simulink model "E33_VCU_simulink"  (R2014a)
settings: Solver=FixedStepDiscrete  StartTime=0.0  StopTime=10.0  FixedStep=0.0005  RelTol=1e-3
values from neighbouring files (symbols this model uses):
  Accu_FAN_Test = ecucoder_cal(Accu_FAN_Test)    [E33_VCU.m]
  Accu_FAN_threshold = ecucoder_cal(Accu_FAN_threshold)    [E33_VCU.m]
  APPS1_Voltage = ecucoder_cal(APPS1_Voltage)    [E33_VCU.m]
  APPS2_Voltage = ecucoder_cal(APPS2_Voltage)    [E33_VCU.m]
  APPS_Map = [0,1000]    [E33_VCU.m]
  APPS_threshold = ecucoder_cal(APPS_threshold)    [E33_VCU.m]
  Beep_Time = ecucoder_cal(Beep_Time)    [E33_VCU.m]
  BeeperTest = ecucoder_cal(BeeperTest)    [E33_VCU.m]
  BMSLedTest = ecucoder_cal(BMSLedTest)    [E33_VCU.m]
  BP_F_threshold = ecucoder_cal(BP_F_threshold)    [E33_VCU.m]
  BP_F_Voltage = ecucoder_cal(BP_F_Voltage)    [E33_VCU.m]
  BP_Map = [0,1000]    [E33_VCU.m]
  BP_R_Voltage = ecucoder_cal(BP_R_Voltage)    [E33_VCU.m]
  Brk_luminance = ecucoder_cal(Brk_luminance)    [E33_VCU.m]
  DCDC_Relay_Test = ecucoder_cal(DCDC_Relay_Test)    [E33_VCU.m]
  FactoryTestEnable = ecucoder_cal(FactoryTestEnable)    [E33_VCU.m]
  HardBrk_luminance = ecucoder_cal(HardBrk_luminance)    [E33_VCU.m]
  IMDLedTest = ecucoder_cal(IMDLedTest)    [E33_VCU.m]
  linear_FL_Map = ecucoder_cal(linear_FL_Map)    [E33_VCU.m]
  linear_FR_Map = ecucoder_cal(linear_FR_Map)    [E33_VCU.m]
  linear_Map = ecucoder_cal(linear_Map)    [E33_VCU.m]
  linear_RL_Map = ecucoder_cal(linear_RL_Map)    [E33_VCU.m]
  linear_RR_Map = ecucoder_cal(linear_RR_Map)    [E33_VCU.m]
  MaxPow = 40    [E33_VCU.m]
  MaxRPM = 5400    [E33_VCU.m]
  MaxRPMchangePerSec = ecucoder_cal(MaxRPMchangePerSec)    [E33_VCU.m]
  MaxTorqChangePerSec = ecucoder_cal(MaxTorqChangePerSec)    [E33_VCU.m]
  Motor_RPM_Map = (0:ceil(MaxRPM/100))*100    [E33_VCU.m]
  Pump_Test = ecucoder_cal(Pump_Test)    [E33_VCU.m]
  Pump_threshold = ecucoder_cal(Pump_threshold)    [E33_VCU.m]
  R2D_Light_Test = ecucoder_cal(R2D_Light_Test)    [E33_VCU.m]
  Radiator_FAN_Test = ecucoder_cal(Radiator_FAN_Test)    [E33_VCU.m]
  SCS_Error_5V = ecucoder_cal(SCS_Error_5V)    [E33_VCU.m]
  SCS_Error_GND = ecucoder_cal(SCS_Error_GND)    [E33_VCU.m]
  SPD_Coef = 1884/40    (= 47.1)    [E33_VCU.m]
  Tail_Light_Test = ecucoder_cal(Tail_Light_Test)    [E33_VCU.m]
  Tmanage_Map = [0,100]    [E33_VCU.m]
  Torq_percentage_Map = Motor_Torq_MAP/MaxTorq*1000    [E33_VCU.m]
libraries: simulink x164, ec55xxlib x44, dspswit3 x6
(part 3 of 5)

== system E33_VCU_simulink/Subsystem1/MCUctrl/VCU_MCU_CMD/MCU_SPD_CMD ==
  MCU_SPD_CMD : Inport
  BitCov : DataTypeConversion  OutDataTypeStr=uint8
  Constant{3..8} (6 alike) : Constant  Value=0  OutDataTypeStr=uint8  SampleTime=-1
  MCU_SPD_CMDCOV : DataTypeConversion  OutDataTypeStr=uint8
  MCU_SPD_CMDRon : Rounding  Operator=round
  MCU_SPD_CMD_1sat : Saturate  UpperLimit=65535  LowerLimit=0
  MCU_SPD_CMD_And : simulink/Logic and Bit Operations/Bitwise Operator  logicop=AND  UseBitMask=off  NumInputPorts=2  BitMask=bin2dec('11011001')  BitMaskRealWorld=Stored Integer
  MCU_SPD_CMD_And_C : Constant  Value=255  OutDataTypeStr=uint32
  MCU_SPD_CMD_Convert : DataTypeConversion  OutDataTypeStr=uint32
  MCU_SPD_CMD_D : Product  Inputs=*/
  MCU_SPD_CMD_D1 : Product  Inputs=*/
  MCU_SPD_CMD_F : Constant  Value=0.5  OutDataTypeStr=single
  MCU_SPD_CMD_L : simulink/Logic and Bit Operations/Bitwise Operator  logicop=AND  UseBitMask=on  BitMask=65535  BitMaskRealWorld=Stored Integer
  MCU_SPD_CMD_O : Constant  Value=-10000  OutDataTypeStr=single
  MCU_SPD_CMD_S : ArithShift
  MCU_SPD_CMD_sat : Saturate  UpperLimit=10000  LowerLimit=-10000
  MCU_SPD_CMD_st : Sum  Inputs=+-
  MCU_SPD_CMDoutput2_C : Constant  Value=256
  output1 : Outport
  output2 : Outport  Port=2
  output3 : Outport  Port=3
  output4 : Outport  Port=4
  output5 : Outport  Port=5
  output6 : Outport  Port=6
  output7 : Outport  Port=7
  output8 : Outport  Port=8
  wires:
  MCU_SPD_CMD/1 -> MCU_SPD_CMD_sat/1
  MCU_SPD_CMD_sat/1 -> MCU_SPD_CMD_st/1
  MCU_SPD_CMD_O/1 -> MCU_SPD_CMD_st/2
  MCU_SPD_CMD_st/1 -> MCU_SPD_CMD_D/1
  MCU_SPD_CMD_F/1 -> MCU_SPD_CMD_D/2
  MCU_SPD_CMD_D/1 -> MCU_SPD_CMDRon/1
  MCU_SPD_CMDRon/1 -> MCU_SPD_CMD_S/1
  MCU_SPD_CMD_S/1 -> MCU_SPD_CMD_1sat/1
  MCU_SPD_CMD_1sat/1 -> MCU_SPD_CMD_Convert/1
  MCU_SPD_CMD_Convert/1 -> MCU_SPD_CMD_L/1
  MCU_SPD_CMD_L/1 -> MCU_SPD_CMD_D1/1, MCU_SPD_CMD_And/1
  MCU_SPD_CMDoutput2_C/1 -> MCU_SPD_CMD_D1/2
  MCU_SPD_CMD_D1/1 -> MCU_SPD_CMDCOV/1
  MCU_SPD_CMDCOV/1 -> output2/1
  MCU_SPD_CMD_And_C/1 -> MCU_SPD_CMD_And/2
  MCU_SPD_CMD_And/1 -> BitCov/1
  BitCov/1 -> output1/1
  Constant3/1 -> output3/1
  Constant4/1 -> output4/1
  Constant5/1 -> output5/1
  Constant6/1 -> output6/1
  Constant7/1 -> output7/1
  Constant8/1 -> output8/1

== system E33_VCU_simulink/Subsystem1/MCUctrl/VCU_MCU_CMD/MCU_TORQ_CMD ==
  MCU_TORQ_CMD : Inport
  BitCov : DataTypeConversion  OutDataTypeStr=uint8
  Constant{1..2,5..8} (6 alike) : Constant  Value=0  OutDataTypeStr=uint8  SampleTime=-1
  MCU_TORQ_CMDCOV : DataTypeConversion  OutDataTypeStr=uint8
  MCU_TORQ_CMDRon : Rounding  Operator=round
  MCU_TORQ_CMD_1sat : Saturate  UpperLimit=65535  LowerLimit=0
  MCU_TORQ_CMD_And : simulink/Logic and Bit Operations/Bitwise Operator  logicop=AND  UseBitMask=off  NumInputPorts=2  BitMask=bin2dec('11011001')  BitMaskRealWorld=Stored Integer
  MCU_TORQ_CMD_And_C : Constant  Value=255  OutDataTypeStr=uint32
  MCU_TORQ_CMD_Convert : DataTypeConversion  OutDataTypeStr=uint32
  MCU_TORQ_CMD_D : Product  Inputs=*/
  MCU_TORQ_CMD_D1 : Product  Inputs=*/
  MCU_TORQ_CMD_F : Constant  OutDataTypeStr=single
  MCU_TORQ_CMD_L : simulink/Logic and Bit Operations/Bitwise Operator  logicop=AND  UseBitMask=on  BitMask=65535  BitMaskRealWorld=Stored Integer
  MCU_TORQ_CMD_O : Constant  Value=0  OutDataTypeStr=single
  MCU_TORQ_CMD_S : ArithShift
  MCU_TORQ_CMD_sat : Saturate  UpperLimit=1000  LowerLimit=0
  MCU_TORQ_CMD_st : Sum  Inputs=+-
  MCU_TORQ_CMDoutput4_C : Constant  Value=256
  output1 : Outport
  output2 : Outport  Port=2
  output3 : Outport  Port=3
  output4 : Outport  Port=4
  output5 : Outport  Port=5
  output6 : Outport  Port=6
  output7 : Outport  Port=7
  output8 : Outport  Port=8
  wires:
  MCU_TORQ_CMD/1 -> MCU_TORQ_CMD_sat/1
  MCU_TORQ_CMD_sat/1 -> MCU_TORQ_CMD_st/1
  MCU_TORQ_CMD_O/1 -> MCU_TORQ_CMD_st/2
  MCU_TORQ_CMD_st/1 -> MCU_TORQ_CMD_D/1
  MCU_TORQ_CMD_F/1 -> MCU_TORQ_CMD_D/2
  MCU_TORQ_CMD_D/1 -> MCU_TORQ_CMDRon/1
  MCU_TORQ_CMDRon/1 -> MCU_TORQ_CMD_S/1
  MCU_TORQ_CMD_S/1 -> MCU_TORQ_CMD_1sat/1
  MCU_TORQ_CMD_1sat/1 -> MCU_TORQ_CMD_Convert/1
  MCU_TORQ_CMD_Convert/1 -> MCU_TORQ_CMD_L/1
  MCU_TORQ_CMD_L/1 -> MCU_TORQ_CMD_D1/1, MCU_TORQ_CMD_And/1
  MCU_TORQ_CMDoutput4_C/1 -> MCU_TORQ_CMD_D1/2
  MCU_TORQ_CMD_D1/1 -> MCU_TORQ_CMDCOV/1
  MCU_TORQ_CMDCOV/1 -> output4/1
  MCU_TORQ_CMD_And_C/1 -> MCU_TORQ_CMD_And/2
  MCU_TORQ_CMD_And/1 -> BitCov/1
  BitCov/1 -> output3/1
  Constant1/1 -> output1/1
  Constant2/1 -> output2/1
  Constant5/1 -> output5/1
  Constant6/1 -> output6/1
  Constant7/1 -> output7/1
  Constant8/1 -> output8/1

== system E33_VCU_simulink/Subsystem1/VCUCAN/VCU_Panel/Linear_FL ==
  Linear_FL : Inport
  Constant{2..8} (7 alike) : Constant  Value=0  OutDataTypeStr=uint8  SampleTime=-1
  Linear_FLABS : Abs
  Linear_FLCS : ArithShift  BitShiftNumber=-8
  Linear_FLConS : Constant  OutDataTypeStr=single
  Linear_FLCosR : Constant  Value=0  OutDataTypeStr=uint8
  Linear_FLROP : RelationalOperator  Operator=<  OutDataTypeStr=boolean
  Linear_FLRon : Rounding  Operator=round
  Linear_FLSW : Switch  Criteria=u2 ~= 0
  Linear_FL_1sat : Saturate  UpperLimit=255  LowerLimit=0
  Linear_FL_Convert : DataTypeConversion  OutDataTypeStr=uint8
  Linear_FL_Convert1 : DataTypeConversion  OutDataTypeStr=uint32
  Linear_FL_D : Product  Inputs=*/
  Linear_FL_F : Constant  OutDataTypeStr=single
  Linear_FL_L : simulink/Logic and Bit Operations/Bitwise Operator  logicop=AND  UseBitMask=on  BitMask=255  BitMaskRealWorld=Stored Integer
  Linear_FL_O : Constant  Value=0  OutDataTypeStr=single
  Linear_FL_S : ArithShift
  Linear_FL_sat : Saturate  UpperLimit=5000  LowerLimit=0
  Linear_FL_st : Sum  Inputs=+-
  Linear_FLsubcon : Sum  Inputs=+-
  output1 : Outport
  output2 : Outport  Port=2
  output3 : Outport  Port=3
  output4 : Outport  Port=4
  output5 : Outport  Port=5
  output6 : Outport  Port=6
  output7 : Outport  Port=7
  output8 : Outport  Port=8
  wires:
  Linear_FL/1 -> Linear_FL_sat/1
  Linear_FL_sat/1 -> Linear_FL_st/1
  Linear_FL_O/1 -> Linear_FL_st/2
  Linear_FL_st/1 -> Linear_FL_D/1
  Linear_FL_F/1 -> Linear_FL_D/2
  Linear_FL_D/1 -> Linear_FLRon/1
  Linear_FLRon/1 -> Linear_FLROP/1, Linear_FLABS/1, Linear_FLSW/3
  Linear_FLCosR/1 -> Linear_FLROP/2
  Linear_FLConS/1 -> Linear_FLCS/1
  Linear_FLCS/1 -> Linear_FLsubcon/1
  Linear_FLABS/1 -> Linear_FLsubcon/2
  Linear_FLsubcon/1 -> Linear_FLSW/1
  Linear_FLROP/1 -> Linear_FLSW/2
  Linear_FLSW/1 -> Linear_FL_S/1
  Linear_FL_S/1 -> Linear_FL_1sat/1
  Linear_FL_1sat/1 -> Linear_FL_Convert1/1
  Linear_FL_Convert1/1 -> Linear_FL_L/1
  Linear_FL_L/1 -> Linear_FL_Convert/1
  Linear_FL_Convert/1 -> output1/1
  Constant2/1 -> output2/1
  Constant3/1 -> output3/1
  Constant4/1 -> output4/1
  Constant5/1 -> output5/1
  Constant6/1 -> output6/1
  Constant7/1 -> output7/1
  Constant8/1 -> output8/1

== system E33_VCU_simulink/Subsystem1/VCUCAN/VCU_Panel/Linear_FR ==
  Linear_FR : Inport
  Constant{1..2,4..8} (7 alike) : Constant  Value=0  OutDataTypeStr=uint8  SampleTime=-1
  Linear_FRABS : Abs
  Linear_FRCS : ArithShift  BitShiftNumber=-8
  Linear_FRConS : Constant  OutDataTypeStr=single
  Linear_FRCosR : Constant  Value=0  OutDataTypeStr=uint8
  Linear_FRROP : RelationalOperator  Operator=<  OutDataTypeStr=boolean
  Linear_FRRon : Rounding  Operator=round
  Linear_FRSW : Switch  Criteria=u2 ~= 0
  Linear_FR_1sat : Saturate  UpperLimit=255  LowerLimit=0
  Linear_FR_Convert : DataTypeConversion  OutDataTypeStr=uint8
  Linear_FR_Convert1 : DataTypeConversion  OutDataTypeStr=uint32
  Linear_FR_D : Product  Inputs=*/
  Linear_FR_F : Constant  OutDataTypeStr=single
  Linear_FR_L : simulink/Logic and Bit Operations/Bitwise Operator  logicop=AND  UseBitMask=on  BitMask=255  BitMaskRealWorld=Stored Integer
  Linear_FR_O : Constant  Value=0  OutDataTypeStr=single
  Linear_FR_S : ArithShift
  Linear_FR_sat : Saturate  UpperLimit=5000  LowerLimit=0
  Linear_FR_st : Sum  Inputs=+-
  Linear_FRsubcon : Sum  Inputs=+-
  output1 : Outport
  output2 : Outport  Port=2
  output3 : Outport  Port=3
  output4 : Outport  Port=4
  output5 : Outport  Port=5
  output6 : Outport  Port=6
  output7 : Outport  Port=7
  output8 : Outport  Port=8
  wires:
  Linear_FR/1 -> Linear_FR_sat/1
  Linear_FR_sat/1 -> Linear_FR_st/1
  Linear_FR_O/1 -> Linear_FR_st/2
  Linear_FR_st/1 -> Linear_FR_D/1
  Linear_FR_F/1 -> Linear_FR_D/2
  Linear_FR_D/1 -> Linear_FRRon/1
  Linear_FRRon/1 -> Linear_FRROP/1, Linear_FRABS/1, Linear_FRSW/3
  Linear_FRCosR/1 -> Linear_FRROP/2
  Linear_FRConS/1 -> Linear_FRCS/1
  Linear_FRCS/1 -> Linear_FRsubcon/1
  Linear_FRABS/1 -> Linear_FRsubcon/2
  Linear_FRsubcon/1 -> Linear_FRSW/1
  Linear_FRROP/1 -> Linear_FRSW/2
  Linear_FRSW/1 -> Linear_FR_S/1
  Linear_FR_S/1 -> Linear_FR_1sat/1
  Linear_FR_1sat/1 -> Linear_FR_Convert1/1
  Linear_FR_Convert1/1 -> Linear_FR_L/1
  Linear_FR_L/1 -> Linear_FR_Convert/1
  Linear_FR_Convert/1 -> output3/1
  Constant1/1 -> output1/1
  Constant2/1 -> output2/1
  Constant4/1 -> output4/1
  Constant5/1 -> output5/1
  Constant6/1 -> output6/1
  Constant7/1 -> output7/1
  Constant8/1 -> output8/1

== system E33_VCU_simulink/Subsystem1/VCUCAN/VCU_Panel/Linear_RL ==
  Linear_RL : Inport
  Constant{1,3..8} (7 alike) : Constant  Value=0  OutDataTypeStr=uint8  SampleTime=-1
  Linear_RLABS : Abs
  Linear_RLCS : ArithShift  BitShiftNumber=-8
  Linear_RLConS : Constant  OutDataTypeStr=single
  Linear_RLCosR : Constant  Value=0  OutDataTypeStr=uint8
  Linear_RLROP : RelationalOperator  Operator=<  OutDataTypeStr=boolean
  Linear_RLRon : Rounding  Operator=round
  Linear_RLSW : Switch  Criteria=u2 ~= 0
  Linear_RL_1sat : Saturate  UpperLimit=255  LowerLimit=0
  Linear_RL_Convert : DataTypeConversion  OutDataTypeStr=uint8
  Linear_RL_Convert1 : DataTypeConversion  OutDataTypeStr=uint32
  Linear_RL_D : Product  Inputs=*/
  Linear_RL_F : Constant  OutDataTypeStr=single
  Linear_RL_L : simulink/Logic and Bit Operations/Bitwise Operator  logicop=AND  UseBitMask=on  BitMask=255  BitMaskRealWorld=Stored Integer
  Linear_RL_O : Constant  Value=0  OutDataTypeStr=single
  Linear_RL_S : ArithShift
  Linear_RL_sat : Saturate  UpperLimit=5000  LowerLimit=0
  Linear_RL_st : Sum  Inputs=+-
  Linear_RLsubcon : Sum  Inputs=+-
  output1 : Outport
  output2 : Outport  Port=2
  output3 : Outport  Port=3
  output4 : Outport  Port=4
  output5 : Outport  Port=5
  output6 : Outport  Port=6
  output7 : Outport  Port=7
  output8 : Outport  Port=8
  wires:
  Linear_RL/1 -> Linear_RL_sat/1
  Linear_RL_sat/1 -> Linear_RL_st/1
  Linear_RL_O/1 -> Linear_RL_st/2
  Linear_RL_st/1 -> Linear_RL_D/1
  Linear_RL_F/1 -> Linear_RL_D/2
  Linear_RL_D/1 -> Linear_RLRon/1
  Linear_RLRon/1 -> Linear_RLROP/1, Linear_RLABS/1, Linear_RLSW/3
  Linear_RLCosR/1 -> Linear_RLROP/2
  Linear_RLConS/1 -> Linear_RLCS/1
  Linear_RLCS/1 -> Linear_RLsubcon/1
  Linear_RLABS/1 -> Linear_RLsubcon/2
  Linear_RLsubcon/1 -> Linear_RLSW/1
  Linear_RLROP/1 -> Linear_RLSW/2
  Linear_RLSW/1 -> Linear_RL_S/1
  Linear_RL_S/1 -> Linear_RL_1sat/1
  Linear_RL_1sat/1 -> Linear_RL_Convert1/1
  Linear_RL_Convert1/1 -> Linear_RL_L/1
  Linear_RL_L/1 -> Linear_RL_Convert/1
  Linear_RL_Convert/1 -> output2/1
  Constant1/1 -> output1/1
  Constant3/1 -> output3/1
  Constant4/1 -> output4/1
  Constant5/1 -> output5/1
  Constant6/1 -> output6/1
  Constant7/1 -> output7/1
  Constant8/1 -> output8/1

== system E33_VCU_simulink/Subsystem1/VCUCAN/VCU_Panel/Linear_RR ==
  Linear_RR : Inport
  Constant{1..3,5..8} (7 alike) : Constant  Value=0  OutDataTypeStr=uint8  SampleTime=-1
  Linear_RRABS : Abs
  Linear_RRCS : ArithShift  BitShiftNumber=-8
  Linear_RRConS : Constant  OutDataTypeStr=single
  Linear_RRCosR : Constant  Value=0  OutDataTypeStr=uint8
  Linear_RRROP : RelationalOperator  Operator=<  OutDataTypeStr=boolean
  Linear_RRRon : Rounding  Operator=round
  Linear_RRSW : Switch  Criteria=u2 ~= 0
  Linear_RR_1sat : Saturate  UpperLimit=255  LowerLimit=0
  Linear_RR_Convert : DataTypeConversion  OutDataTypeStr=uint8
  Linear_RR_Convert1 : DataTypeConversion  OutDataTypeStr=uint32
  Linear_RR_D : Product  Inputs=*/
  Linear_RR_F : Constant  OutDataTypeStr=single
  Linear_RR_L : simulink/Logic and Bit Operations/Bitwise Operator  logicop=AND  UseBitMask=on  BitMask=255  BitMaskRealWorld=Stored Integer
  Linear_RR_O : Constant  Value=0  OutDataTypeStr=single
  Linear_RR_S : ArithShift
  Linear_RR_sat : Saturate  UpperLimit=5000  LowerLimit=0
  Linear_RR_st : Sum  Inputs=+-
  Linear_RRsubcon : Sum  Inputs=+-
  output1 : Outport
  output2 : Outport  Port=2
  output3 : Outport  Port=3
  output4 : Outport  Port=4
  output5 : Outport  Port=5
  output6 : Outport  Port=6
  output7 : Outport  Port=7
  output8 : Outport  Port=8
  wires:
  Linear_RR/1 -> Linear_RR_sat/1
  Linear_RR_sat/1 -> Linear_RR_st/1
  Linear_RR_O/1 -> Linear_RR_st/2
  Linear_RR_st/1 -> Linear_RR_D/1
  Linear_RR_F/1 -> Linear_RR_D/2
  Linear_RR_D/1 -> Linear_RRRon/1
  Linear_RRRon/1 -> Linear_RRROP/1, Linear_RRABS/1, Linear_RRSW/3
  Linear_RRCosR/1 -> Linear_RRROP/2
  Linear_RRConS/1 -> Linear_RRCS/1
  Linear_RRCS/1 -> Linear_RRsubcon/1
  Linear_RRABS/1 -> Linear_RRsubcon/2
  Linear_RRsubcon/1 -> Linear_RRSW/1
  Linear_RRROP/1 -> Linear_RRSW/2
  Linear_RRSW/1 -> Linear_RR_S/1
  Linear_RR_S/1 -> Linear_RR_1sat/1
  Linear_RR_1sat/1 -> Linear_RR_Convert1/1
  Linear_RR_Convert1/1 -> Linear_RR_L/1
  Linear_RR_L/1 -> Linear_RR_Convert/1
  Linear_RR_Convert/1 -> output4/1
  Constant1/1 -> output1/1
  Constant2/1 -> output2/1
  Constant3/1 -> output3/1
  Constant5/1 -> output5/1
  Constant6/1 -> output6/1
  Constant7/1 -> output7/1
  Constant8/1 -> output8/1

== system E33_VCU_simulink/Subsystem1/VCUCAN/VCU_Panel/Wheel_Angle ==
  Wheel_Angle : Inport
  Constant{1..4,6..8} (7 alike) : Constant  Value=0  OutDataTypeStr=uint8  SampleTime=-1
  Wheel_AngleABS : Abs
  Wheel_AngleCS : ArithShift  BitShiftNumber=-8
  Wheel_AngleConS : Constant  OutDataTypeStr=single
  Wheel_AngleCosR : Constant  Value=0  OutDataTypeStr=uint8
  Wheel_AngleROP : RelationalOperator  Operator=<  OutDataTypeStr=boolean
  Wheel_AngleRon : Rounding  Operator=round
  Wheel_AngleSW : Switch  Criteria=u2 ~= 0
  Wheel_Angle_1sat : Saturate  UpperLimit=255  LowerLimit=0
  Wheel_Angle_Convert : DataTypeConversion  OutDataTypeStr=uint8
  Wheel_Angle_Convert1 : DataTypeConversion  OutDataTypeStr=uint32
  Wheel_Angle_D : Product  Inputs=*/
  Wheel_Angle_F : Constant  OutDataTypeStr=single
  Wheel_Angle_L : simulink/Logic and Bit Operations/Bitwise Operator  logicop=AND  UseBitMask=on  BitMask=255  BitMaskRealWorld=Stored Integer
  Wheel_Angle_O : Constant  Value=0  OutDataTypeStr=single
  Wheel_Angle_S : ArithShift
  Wheel_Angle_sat : Saturate  UpperLimit=5000  LowerLimit=0
  Wheel_Angle_st : Sum  Inputs=+-
  Wheel_Anglesubcon : Sum  Inputs=+-
  output1 : Outport
  output2 : Outport  Port=2
  output3 : Outport  Port=3
  output4 : Outport  Port=4
  output5 : Outport  Port=5
  output6 : Outport  Port=6
  output7 : Outport  Port=7
  output8 : Outport  Port=8
  wires:
  Wheel_Angle/1 -> Wheel_Angle_sat/1
  Wheel_Angle_sat/1 -> Wheel_Angle_st/1
  Wheel_Angle_O/1 -> Wheel_Angle_st/2
  Wheel_Angle_st/1 -> Wheel_Angle_D/1
  Wheel_Angle_F/1 -> Wheel_Angle_D/2
  Wheel_Angle_D/1 -> Wheel_AngleRon/1
  Wheel_AngleRon/1 -> Wheel_AngleROP/1, Wheel_AngleABS/1, Wheel_AngleSW/3
  Wheel_AngleCosR/1 -> Wheel_AngleROP/2
  Wheel_AngleConS/1 -> Wheel_AngleCS/1
  Wheel_AngleCS/1 -> Wheel_Anglesubcon/1
  Wheel_AngleABS/1 -> Wheel_Anglesubcon/2
  Wheel_Anglesubcon/1 -> Wheel_AngleSW/1
  Wheel_AngleROP/1 -> Wheel_AngleSW/2
  Wheel_AngleSW/1 -> Wheel_Angle_S/1
  Wheel_Angle_S/1 -> Wheel_Angle_1sat/1
  Wheel_Angle_1sat/1 -> Wheel_Angle_Convert1/1
  Wheel_Angle_Convert1/1 -> Wheel_Angle_L/1
  Wheel_Angle_L/1 -> Wheel_Angle_Convert/1
  Wheel_Angle_Convert/1 -> output5/1
  Constant1/1 -> output1/1
  Constant2/1 -> output2/1
  Constant3/1 -> output3/1
  Constant4/1 -> output4/1
  Constant6/1 -> output6/1
  Constant7/1 -> output7/1
  Constant8/1 -> output8/1

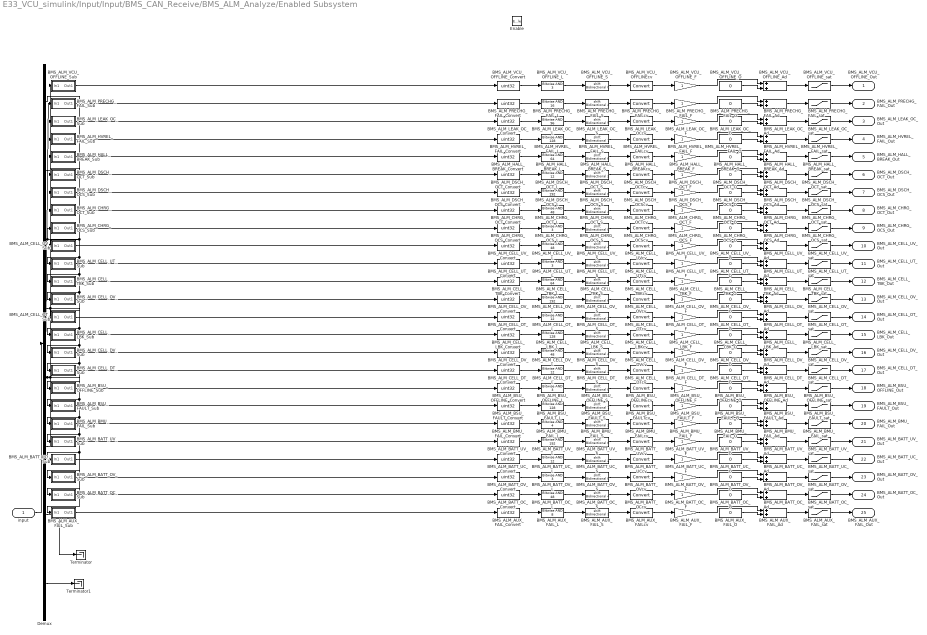
== system E33_VCU_simulink/Input/Input/BMS_CAN_Receive/BMS_ALM_Analyze/Enabled Subsystem ==
  input : Inport
  Enable : EnablePort
  BMS_ALM_AUX_FAIL_Ad : Sum
  BMS_ALM_AUX_FAIL_Convert : DataTypeConversion  OutDataTypeStr=uint32
  BMS_ALM_AUX_FAIL_F : Gain
  BMS_ALM_AUX_FAIL_L : simulink/Logic and Bit Operations/Bitwise Operator  logicop=AND  UseBitMask=on  BitMask=8  BitMaskRealWorld=Stored Integer
  BMS_ALM_AUX_FAIL_O : Constant  Value=0  OutDataTypeStr=single
  BMS_ALM_AUX_FAIL_S : ArithShift  BitShiftNumber=3
  BMS_ALM_AUX_FAIL_Sub : Subsystem
  BMS_ALM_AUX_FAIL_sat : Saturate  UpperLimit=3  LowerLimit=0
  BMS_ALM_AUX_FAILcv : DataTypeConversion
  BMS_ALM_BATT_OC_Ad : Sum
  BMS_ALM_BATT_OC_Convert : DataTypeConversion  OutDataTypeStr=uint32
  BMS_ALM_BATT_OC_F : Gain
  BMS_ALM_BATT_OC_L : simulink/Logic and Bit Operations/Bitwise Operator  logicop=AND  UseBitMask=on  BitMask=48  BitMaskRealWorld=Stored Integer
  BMS_ALM_BATT_OC_O : Constant  Value=0  OutDataTypeStr=single
  BMS_ALM_BATT_OC_S : ArithShift  BitShiftNumber=4
  BMS_ALM_BATT_OC_Sub : Subsystem
  BMS_ALM_BATT_OC_sat : Saturate  UpperLimit=3  LowerLimit=0
  BMS_ALM_BATT_OCcv : DataTypeConversion
  BMS_ALM_BATT_OV_Ad : Sum
  BMS_ALM_BATT_OV_Convert : DataTypeConversion  OutDataTypeStr=uint32
  BMS_ALM_BATT_OV_F : Gain
  BMS_ALM_BATT_OV_L : simulink/Logic and Bit Operations/Bitwise Operator  logicop=AND  UseBitMask=on  BitMask=3  BitMaskRealWorld=Stored Integer
  BMS_ALM_BATT_OV_O : Constant  Value=0  OutDataTypeStr=single
  BMS_ALM_BATT_OV_S : ArithShift
  BMS_ALM_BATT_OV_Sub : Subsystem
  BMS_ALM_BATT_OV_sat : Saturate  UpperLimit=3  LowerLimit=0
  BMS_ALM_BATT_OVcv : DataTypeConversion
  BMS_ALM_BATT_UC_Ad : Sum
  BMS_ALM_BATT_UC_Convert : DataTypeConversion  OutDataTypeStr=uint32
  BMS_ALM_BATT_UC_F : Gain
  BMS_ALM_BATT_UC_L : simulink/Logic and Bit Operations/Bitwise Operator  logicop=AND  UseBitMask=on  BitMask=12  BitMaskRealWorld=Stored Integer
  BMS_ALM_BATT_UC_O : Constant  Value=0  OutDataTypeStr=single
  BMS_ALM_BATT_UC_S : ArithShift  BitShiftNumber=2
  BMS_ALM_BATT_UC_Sub : Subsystem
  BMS_ALM_BATT_UC_sat : Saturate  UpperLimit=3  LowerLimit=0
  BMS_ALM_BATT_UCcv : DataTypeConversion
  BMS_ALM_BATT_UV_Ad : Sum
  BMS_ALM_BATT_UV_Convert : DataTypeConversion  OutDataTypeStr=uint32
  BMS_ALM_BATT_UV_F : Gain
  BMS_ALM_BATT_UV_L : simulink/Logic and Bit Operations/Bitwise Operator  logicop=AND  UseBitMask=on  BitMask=192  BitMaskRealWorld=Stored Integer
  BMS_ALM_BATT_UV_O : Constant  Value=0  OutDataTypeStr=single
  BMS_ALM_BATT_UV_S : ArithShift  BitShiftNumber=6
  BMS_ALM_BATT_UV_Sub : Subsystem
  BMS_ALM_BATT_UV_sat : Saturate  UpperLimit=3  LowerLimit=0
  BMS_ALM_BATT_UVcv : DataTypeConversion
  BMS_ALM_BMU_FAIL_Ad : Sum
  BMS_ALM_BMU_FAIL_Convert : DataTypeConversion  OutDataTypeStr=uint32
  BMS_ALM_BMU_FAIL_F : Gain
  BMS_ALM_BMU_FAIL_L : simulink/Logic and Bit Operations/Bitwise Operator  logicop=AND  UseBitMask=on  BitMask=4  BitMaskRealWorld=Stored Integer
  BMS_ALM_BMU_FAIL_O : Constant  Value=0  OutDataTypeStr=single
  BMS_ALM_BMU_FAIL_S : ArithShift  BitShiftNumber=2
  BMS_ALM_BMU_FAIL_Sub : Subsystem
  BMS_ALM_BMU_FAIL_sat : Saturate  UpperLimit=3  LowerLimit=0
  BMS_ALM_BMU_FAILcv : DataTypeConversion
  BMS_ALM_BSU_FAULT_Ad : Sum
  BMS_ALM_BSU_FAULT_Convert : DataTypeConversion  OutDataTypeStr=uint32
  BMS_ALM_BSU_FAULT_F : Gain
  BMS_ALM_BSU_FAULT_L : simulink/Logic and Bit Operations/Bitwise Operator  logicop=AND  UseBitMask=on  BitMask=128  BitMaskRealWorld=Stored Integer
  BMS_ALM_BSU_FAULT_O : Constant  Value=0  OutDataTypeStr=single
  BMS_ALM_BSU_FAULT_S : ArithShift  BitShiftNumber=7
  BMS_ALM_BSU_FAULT_Sub : Subsystem
  BMS_ALM_BSU_FAULT_sat : Saturate  UpperLimit=3  LowerLimit=0
  BMS_ALM_BSU_FAULTcv : DataTypeConversion
  BMS_ALM_BSU_OFFLINE_Ad : Sum
  BMS_ALM_BSU_OFFLINE_Convert : DataTypeConversion  OutDataTypeStr=uint32
  BMS_ALM_BSU_OFFLINE_F : Gain
  BMS_ALM_BSU_OFFLINE_L : simulink/Logic and Bit Operations/Bitwise Operator  logicop=AND  UseBitMask=on  BitMask=3  BitMaskRealWorld=Stored Integer
  BMS_ALM_BSU_OFFLINE_O : Constant  Value=0  OutDataTypeStr=single
  BMS_ALM_BSU_OFFLINE_S : ArithShift
  BMS_ALM_BSU_OFFLINE_Sub : Subsystem
  BMS_ALM_BSU_OFFLINE_sat : Saturate  UpperLimit=3  LowerLimit=0
  BMS_ALM_BSU_OFFLINEcv : DataTypeConversion
  BMS_ALM_CELL_DT_Ad : Sum
  BMS_ALM_CELL_DT_Convert : DataTypeConversion  OutDataTypeStr=uint32
  BMS_ALM_CELL_DT_F : Gain
  BMS_ALM_CELL_DT_L : simulink/Logic and Bit Operations/Bitwise Operator  logicop=AND  UseBitMask=on  BitMask=12  BitMaskRealWorld=Stored Integer
  BMS_ALM_CELL_DT_O : Constant  Value=0  OutDataTypeStr=single
  BMS_ALM_CELL_DT_S : ArithShift  BitShiftNumber=2
  BMS_ALM_CELL_DT_Sub : Subsystem
  BMS_ALM_CELL_DT_sat : Saturate  UpperLimit=3  LowerLimit=0
  BMS_ALM_CELL_DTcv : DataTypeConversion
  BMS_ALM_CELL_DV_Ad : Sum
  BMS_ALM_CELL_DV_Convert : DataTypeConversion  OutDataTypeStr=uint32
  BMS_ALM_CELL_DV_F : Gain
  BMS_ALM_CELL_DV_L : simulink/Logic and Bit Operations/Bitwise Operator  logicop=AND  UseBitMask=on  BitMask=48  BitMaskRealWorld=Stored Integer
  BMS_ALM_CELL_DV_O : Constant  Value=0  OutDataTypeStr=single
  BMS_ALM_CELL_DV_S : ArithShift  BitShiftNumber=4
  BMS_ALM_CELL_DV_Sub : Subsystem
  BMS_ALM_CELL_DV_sat : Saturate  UpperLimit=3  LowerLimit=0
  BMS_ALM_CELL_DVcv : DataTypeConversion
  BMS_ALM_CELL_LBK_Ad : Sum
  BMS_ALM_CELL_LBK_Convert : DataTypeConversion  OutDataTypeStr=uint32
  BMS_ALM_CELL_LBK_F : Gain
  BMS_ALM_CELL_LBK_L : simulink/Logic and Bit Operations/Bitwise Operator  logicop=AND  UseBitMask=on  BitMask=128  BitMaskRealWorld=Stored Integer
  BMS_ALM_CELL_LBK_O : Constant  Value=0  OutDataTypeStr=single
  BMS_ALM_CELL_LBK_S : ArithShift  BitShiftNumber=7
  BMS_ALM_CELL_LBK_Sub : Subsystem
  BMS_ALM_CELL_LBK_sat : Saturate  UpperLimit=3  LowerLimit=0
  BMS_ALM_CELL_LBKcv : DataTypeConversion
  BMS_ALM_CELL_OT_Ad : Sum
  BMS_ALM_CELL_OT_Convert : DataTypeConversion  OutDataTypeStr=uint32
  BMS_ALM_CELL_OT_F : Gain
  BMS_ALM_CELL_OT_L : simulink/Logic and Bit Operations/Bitwise Operator  logicop=AND  UseBitMask=on  BitMask=12  BitMaskRealWorld=Stored Integer
  BMS_ALM_CELL_OT_O : Constant  Value=0  OutDataTypeStr=single
  BMS_ALM_CELL_OT_S : ArithShift  BitShiftNumber=2
  BMS_ALM_CELL_OT_Sub : Subsystem
  BMS_ALM_CELL_OT_sat : Saturate  UpperLimit=3  LowerLimit=0
  BMS_ALM_CELL_OTcv : DataTypeConversion
  BMS_ALM_CELL_OV_Ad : Sum
  BMS_ALM_CELL_OV_Convert : DataTypeConversion  OutDataTypeStr=uint32
  BMS_ALM_CELL_OV_F : Gain
  BMS_ALM_CELL_OV_L : simulink/Logic and Bit Operations/Bitwise Operator  logicop=AND  UseBitMask=on  BitMask=192  BitMaskRealWorld=Stored Integer
  BMS_ALM_CELL_OV_O : Constant  Value=0  OutDataTypeStr=single
  BMS_ALM_CELL_OV_S : ArithShift  BitShiftNumber=6
  BMS_ALM_CELL_OV_Sub : Subsystem
  BMS_ALM_CELL_OV_sat : Saturate  UpperLimit=3  LowerLimit=0
  BMS_ALM_CELL_OVcv : DataTypeConversion
  BMS_ALM_CELL_TBK_Ad : Sum
  BMS_ALM_CELL_TBK_Convert : DataTypeConversion  OutDataTypeStr=uint32
  BMS_ALM_CELL_TBK_F : Gain
  BMS_ALM_CELL_TBK_L : simulink/Logic and Bit Operations/Bitwise Operator  logicop=AND  UseBitMask=on  BitMask=64  BitMaskRealWorld=Stored Integer
  BMS_ALM_CELL_TBK_O : Constant  Value=0  OutDataTypeStr=single
  BMS_ALM_CELL_TBK_S : ArithShift  BitShiftNumber=6
  BMS_ALM_CELL_TBK_Sub : Subsystem
  BMS_ALM_CELL_TBK_sat : Saturate  UpperLimit=3  LowerLimit=0
  BMS_ALM_CELL_TBKcv : DataTypeConversion
  BMS_ALM_CELL_UT_Ad : Sum
  BMS_ALM_CELL_UT_Convert : DataTypeConversion  OutDataTypeStr=uint32
  BMS_ALM_CELL_UT_F : Gain
  BMS_ALM_CELL_UT_L : simulink/Logic and Bit Operations/Bitwise Operator  logicop=AND  UseBitMask=on  BitMask=3  BitMaskRealWorld=Stored Integer
  BMS_ALM_CELL_UT_O : Constant  Value=0  OutDataTypeStr=single
  BMS_ALM_CELL_UT_S : ArithShift
  BMS_ALM_CELL_UT_Sub : Subsystem
  BMS_ALM_CELL_UT_sat : Saturate  UpperLimit=3  LowerLimit=0
  BMS_ALM_CELL_UTcv : DataTypeConversion
  BMS_ALM_CELL_UV_Ad : Sum
  BMS_ALM_CELL_UV_Convert : DataTypeConversion  OutDataTypeStr=uint32
  BMS_ALM_CELL_UV_F : Gain
  BMS_ALM_CELL_UV_L : simulink/Logic and Bit Operations/Bitwise Operator  logicop=AND  UseBitMask=on  BitMask=48  BitMaskRealWorld=Stored Integer
  BMS_ALM_CELL_UV_O : Constant  Value=0  OutDataTypeStr=single
  BMS_ALM_CELL_UV_S : ArithShift  BitShiftNumber=4
  BMS_ALM_CELL_UV_Sub : Subsystem
  BMS_ALM_CELL_UV_sat : Saturate  UpperLimit=3  LowerLimit=0
  BMS_ALM_CELL_UVcv : DataTypeConversion
  BMS_ALM_CHRG_OCS_Ad : Sum
  BMS_ALM_CHRG_OCS_Convert : DataTypeConversion  OutDataTypeStr=uint32
  BMS_ALM_CHRG_OCS_F : Gain
  BMS_ALM_CHRG_OCS_L : simulink/Logic and Bit Operations/Bitwise Operator  logicop=AND  UseBitMask=on  BitMask=3  BitMaskRealWorld=Stored Integer
  BMS_ALM_CHRG_OCS_O : Constant  Value=0  OutDataTypeStr=single
  BMS_ALM_CHRG_OCS_S : ArithShift
  BMS_ALM_CHRG_OCS_Sub : Subsystem
  BMS_ALM_CHRG_OCS_sat : Saturate  UpperLimit=3  LowerLimit=0
  BMS_ALM_CHRG_OCScv : DataTypeConversion
  BMS_ALM_CHRG_OCT_Ad : Sum
  BMS_ALM_CHRG_OCT_Convert : DataTypeConversion  OutDataTypeStr=uint32
  BMS_ALM_CHRG_OCT_F : Gain
  BMS_ALM_CHRG_OCT_L : simulink/Logic and Bit Operations/Bitwise Operator  logicop=AND  UseBitMask=on  BitMask=48  BitMaskRealWorld=Stored Integer
  BMS_ALM_CHRG_OCT_O : Constant  Value=0  OutDataTypeStr=single
  BMS_ALM_CHRG_OCT_S : ArithShift  BitShiftNumber=4
  BMS_ALM_CHRG_OCT_Sub : Subsystem
  BMS_ALM_CHRG_OCT_sat : Saturate  UpperLimit=3  LowerLimit=0
  BMS_ALM_CHRG_OCTcv : DataTypeConversion
  BMS_ALM_DSCH_OCS_Ad : Sum
  BMS_ALM_DSCH_OCS_Convert : DataTypeConversion  OutDataTypeStr=uint32
  BMS_ALM_DSCH_OCS_F : Gain
  BMS_ALM_DSCH_OCS_L : simulink/Logic and Bit Operations/Bitwise Operator  logicop=AND  UseBitMask=on  BitMask=192  BitMaskRealWorld=Stored Integer
  BMS_ALM_DSCH_OCS_O : Constant  Value=0  OutDataTypeStr=single
  BMS_ALM_DSCH_OCS_S : ArithShift  BitShiftNumber=6
  BMS_ALM_DSCH_OCS_Sub : Subsystem
  BMS_ALM_DSCH_OCS_sat : Saturate  UpperLimit=3  LowerLimit=0
  BMS_ALM_DSCH_OCScv : DataTypeConversion
  BMS_ALM_DSCH_OCT_Ad : Sum
  BMS_ALM_DSCH_OCT_Convert : DataTypeConversion  OutDataTypeStr=uint32
  BMS_ALM_DSCH_OCT_F : Gain
  BMS_ALM_DSCH_OCT_L : simulink/Logic and Bit Operations/Bitwise Operator  logicop=AND  UseBitMask=on  BitMask=12  BitMaskRealWorld=Stored Integer
  BMS_ALM_DSCH_OCT_O : Constant  Value=0  OutDataTypeStr=single
  BMS_ALM_DSCH_OCT_S : ArithShift  BitShiftNumber=2
  BMS_ALM_DSCH_OCT_Sub : Subsystem
  BMS_ALM_DSCH_OCT_sat : Saturate  UpperLimit=3  LowerLimit=0
  BMS_ALM_DSCH_OCTcv : DataTypeConversion
  BMS_ALM_HALL_BREAK_Ad : Sum
  BMS_ALM_HALL_BREAK_Convert : DataTypeConversion  OutDataTypeStr=uint32
  BMS_ALM_HALL_BREAK_F : Gain
  BMS_ALM_HALL_BREAK_L : simulink/Logic and Bit Operations/Bitwise Operator  logicop=AND  UseBitMask=on  BitMask=64  BitMaskRealWorld=Stored Integer
  BMS_ALM_HALL_BREAK_O : Constant  Value=0  OutDataTypeStr=single
  BMS_ALM_HALL_BREAK_S : ArithShift  BitShiftNumber=6
  BMS_ALM_HALL_BREAK_Sub : Subsystem
  BMS_ALM_HALL_BREAK_sat : Saturate  UpperLimit=3  LowerLimit=0
  BMS_ALM_HALL_BREAKcv : DataTypeConversion
  BMS_ALM_HVREL_FAIL_Ad : Sum
  BMS_ALM_HVREL_FAIL_Convert : DataTypeConversion  OutDataTypeStr=uint32
  BMS_ALM_HVREL_FAIL_F : Gain
  BMS_ALM_HVREL_FAIL_L : simulink/Logic and Bit Operations/Bitwise Operator  logicop=AND  UseBitMask=on  BitMask=128  BitMaskRealWorld=Stored Integer
  BMS_ALM_HVREL_FAIL_O : Constant  Value=0  OutDataTypeStr=single
  BMS_ALM_HVREL_FAIL_S : ArithShift  BitShiftNumber=7
  BMS_ALM_HVREL_FAIL_Sub : Subsystem
  BMS_ALM_HVREL_FAIL_sat : Saturate  UpperLimit=3  LowerLimit=0
  BMS_ALM_HVREL_FAILcv : DataTypeConversion
  BMS_ALM_LEAK_OC_Ad : Sum
  BMS_ALM_LEAK_OC_Convert : DataTypeConversion  OutDataTypeStr=uint32
  BMS_ALM_LEAK_OC_F : Gain
  BMS_ALM_LEAK_OC_L : simulink/Logic and Bit Operations/Bitwise Operator  logicop=AND  UseBitMask=on  BitMask=96  BitMaskRealWorld=Stored Integer
  BMS_ALM_LEAK_OC_O : Constant  Value=0  OutDataTypeStr=single
  BMS_ALM_LEAK_OC_S : ArithShift  BitShiftNumber=5
  BMS_ALM_LEAK_OC_Sub : Subsystem
  BMS_ALM_LEAK_OC_sat : Saturate  UpperLimit=3  LowerLimit=0
  BMS_ALM_LEAK_OCcv : DataTypeConversion
  BMS_ALM_PRECHG_FAIL_Ad : Sum
  BMS_ALM_PRECHG_FAIL_Convert : DataTypeConversion  OutDataTypeStr=uint32
  BMS_ALM_PRECHG_FAIL_F : Gain
  BMS_ALM_PRECHG_FAIL_L : simulink/Logic and Bit Operations/Bitwise Operator  logicop=AND  UseBitMask=on  BitMask=16  BitMaskRealWorld=Stored Integer
  BMS_ALM_PRECHG_FAIL_O : Constant  Value=0  OutDataTypeStr=single
  BMS_ALM_PRECHG_FAIL_S : ArithShift  BitShiftNumber=4
  BMS_ALM_PRECHG_FAIL_Sub : Subsystem
  BMS_ALM_PRECHG_FAIL_sat : Saturate  UpperLimit=3  LowerLimit=0
  BMS_ALM_PRECHG_FAILcv : DataTypeConversion
  BMS_ALM_VCU_OFFLINE_Ad : Sum
  BMS_ALM_VCU_OFFLINE_Convert : DataTypeConversion  OutDataTypeStr=uint32
  BMS_ALM_VCU_OFFLINE_F : Gain
  BMS_ALM_VCU_OFFLINE_L : simulink/Logic and Bit Operations/Bitwise Operator  logicop=AND  UseBitMask=on  BitMask=3  BitMaskRealWorld=Stored Integer
  BMS_ALM_VCU_OFFLINE_O : Constant  Value=0  OutDataTypeStr=single
  BMS_ALM_VCU_OFFLINE_S : ArithShift
  BMS_ALM_VCU_OFFLINE_Sub : Subsystem
  BMS_ALM_VCU_OFFLINE_sat : Saturate  UpperLimit=3  LowerLimit=0
  BMS_ALM_VCU_OFFLINEcv : DataTypeConversion
  Demux : Demux  Outputs=8
  Terminator : Terminator
  Terminator1 : Terminator
  BMS_ALM_VCU_OFFLINE_Out : Outport
  BMS_ALM_PRECHG_FAIL_Out : Outport  Port=2
  BMS_ALM_LEAK_OC_Out : Outport  Port=3
  BMS_ALM_HVREL_FAIL_Out : Outport  Port=4
  BMS_ALM_HALL_BREAK_Out : Outport  Port=5
  BMS_ALM_DSCH_OCT_Out : Outport  Port=6
  BMS_ALM_DSCH_OCS_Out : Outport  Port=7
  BMS_ALM_CHRG_OCT_Out : Outport  Port=8
  BMS_ALM_CHRG_OCS_Out : Outport  Port=9
  BMS_ALM_CELL_UV_Out : Outport  Port=10
  BMS_ALM_CELL_UT_Out : Outport  Port=11
  BMS_ALM_CELL_TBK_Out : Outport  Port=12
  BMS_ALM_CELL_OV_Out : Outport  Port=13
  BMS_ALM_CELL_OT_Out : Outport  Port=14
  BMS_ALM_CELL_LBK_Out : Outport  Port=15
  BMS_ALM_CELL_DV_Out : Outport  Port=16
  BMS_ALM_CELL_DT_Out : Outport  Port=17
  BMS_ALM_BSU_OFFLINE_Out : Outport  Port=18
  BMS_ALM_BSU_FAULT_Out : Outport  Port=19
  BMS_ALM_BMU_FAIL_Out : Outport  Port=20
  BMS_ALM_BATT_UV_Out : Outport  Port=21
  BMS_ALM_BATT_UC_Out : Outport  Port=22
  BMS_ALM_BATT_OV_Out : Outport  Port=23
  BMS_ALM_BATT_OC_Out : Outport  Port=24
  BMS_ALM_AUX_FAIL_Out : Outport  Port=25
  wires:
  BMS_ALM_VCU_OFFLINE_F/1 -> BMS_ALM_VCU_OFFLINE_Ad/1
  BMS_ALM_VCU_OFFLINE_O/1 -> BMS_ALM_VCU_OFFLINE_Ad/2
  BMS_ALM_VCU_OFFLINE_Ad/1 -> BMS_ALM_VCU_OFFLINE_sat/1
  BMS_ALM_VCU_OFFLINE_sat/1 -> BMS_ALM_VCU_OFFLINE_Out/1
  Demux/5 -> BMS_ALM_BMU_FAIL_Sub/1(In1), BMS_ALM_AUX_FAIL_Sub/1(In1), BMS_ALM_BSU_FAULT_Sub/1(In1), BMS_ALM_VCU_OFFLINE_Sub/1(In1), BMS_ALM_LEAK_OC_Sub/1(In1), BMS_ALM_PRECHG_FAIL_Sub/1(In1)
  BMS_ALM_VCU_OFFLINE_Sub/1(Out1) -> BMS_ALM_VCU_OFFLINE_Convert/1
  BMS_ALM_VCU_OFFLINE_Convert/1 -> BMS_ALM_VCU_OFFLINE_L/1
  BMS_ALM_VCU_OFFLINE_L/1 -> BMS_ALM_VCU_OFFLINE_S/1
  BMS_ALM_VCU_OFFLINE_S/1 -> BMS_ALM_VCU_OFFLINEcv/1
  BMS_ALM_VCU_OFFLINEcv/1 -> BMS_ALM_VCU_OFFLINE_F/1
  BMS_ALM_PRECHG_FAIL_F/1 -> BMS_ALM_PRECHG_FAIL_Ad/1
  BMS_ALM_PRECHG_FAIL_O/1 -> BMS_ALM_PRECHG_FAIL_Ad/2
  BMS_ALM_PRECHG_FAIL_Ad/1 -> BMS_ALM_PRECHG_FAIL_sat/1
  BMS_ALM_PRECHG_FAIL_sat/1 -> BMS_ALM_PRECHG_FAIL_Out/1
  BMS_ALM_PRECHG_FAIL_Sub/1(Out1) -> BMS_ALM_PRECHG_FAIL_Convert/1
  BMS_ALM_PRECHG_FAIL_Convert/1 -> BMS_ALM_PRECHG_FAIL_L/1
  BMS_ALM_PRECHG_FAIL_L/1 -> BMS_ALM_PRECHG_FAIL_S/1
  BMS_ALM_PRECHG_FAIL_S/1 -> BMS_ALM_PRECHG_FAILcv/1
  BMS_ALM_PRECHG_FAILcv/1 -> BMS_ALM_PRECHG_FAIL_F/1
  BMS_ALM_LEAK_OC_F/1 -> BMS_ALM_LEAK_OC_Ad/1
  BMS_ALM_LEAK_OC_O/1 -> BMS_ALM_LEAK_OC_Ad/2
  BMS_ALM_LEAK_OC_Ad/1 -> BMS_ALM_LEAK_OC_sat/1
  BMS_ALM_LEAK_OC_sat/1 -> BMS_ALM_LEAK_OC_Out/1
  BMS_ALM_LEAK_OC_Sub/1(Out1) -> BMS_ALM_LEAK_OC_Convert/1
  BMS_ALM_LEAK_OC_Convert/1 -> BMS_ALM_LEAK_OC_L/1
  BMS_ALM_LEAK_OC_L/1 -> BMS_ALM_LEAK_OC_S/1
  BMS_ALM_LEAK_OC_S/1 -> BMS_ALM_LEAK_OCcv/1
  BMS_ALM_LEAK_OCcv/1 -> BMS_ALM_LEAK_OC_F/1
  BMS_ALM_HVREL_FAIL_F/1 -> BMS_ALM_HVREL_FAIL_Ad/1
  BMS_ALM_HVREL_FAIL_O/1 -> BMS_ALM_HVREL_FAIL_Ad/2
  BMS_ALM_HVREL_FAIL_Ad/1 -> BMS_ALM_HVREL_FAIL_sat/1
  BMS_ALM_HVREL_FAIL_sat/1 -> BMS_ALM_HVREL_FAIL_Out/1
  Demux/6 -> BMS_ALM_HVREL_FAIL_Sub/1(In1), BMS_ALM_HALL_BREAK_Sub/1(In1)
  BMS_ALM_HVREL_FAIL_Sub/1(Out1) -> BMS_ALM_HVREL_FAIL_Convert/1
  BMS_ALM_HVREL_FAIL_Convert/1 -> BMS_ALM_HVREL_FAIL_L/1
  BMS_ALM_HVREL_FAIL_L/1 -> BMS_ALM_HVREL_FAIL_S/1
  BMS_ALM_HVREL_FAIL_S/1 -> BMS_ALM_HVREL_FAILcv/1
  BMS_ALM_HVREL_FAILcv/1 -> BMS_ALM_HVREL_FAIL_F/1
  BMS_ALM_HALL_BREAK_F/1 -> BMS_ALM_HALL_BREAK_Ad/1
  BMS_ALM_HALL_BREAK_O/1 -> BMS_ALM_HALL_BREAK_Ad/2
  BMS_ALM_HALL_BREAK_Ad/1 -> BMS_ALM_HALL_BREAK_sat/1
  BMS_ALM_HALL_BREAK_sat/1 -> BMS_ALM_HALL_BREAK_Out/1
  BMS_ALM_HALL_BREAK_Sub/1(Out1) -> BMS_ALM_HALL_BREAK_Convert/1
  BMS_ALM_HALL_BREAK_Convert/1 -> BMS_ALM_HALL_BREAK_L/1
  BMS_ALM_HALL_BREAK_L/1 -> BMS_ALM_HALL_BREAK_S/1
  BMS_ALM_HALL_BREAK_S/1 -> BMS_ALM_HALL_BREAKcv/1
  BMS_ALM_HALL_BREAKcv/1 -> BMS_ALM_HALL_BREAK_F/1
  BMS_ALM_DSCH_OCT_F/1 -> BMS_ALM_DSCH_OCT_Ad/1
  BMS_ALM_DSCH_OCT_O/1 -> BMS_ALM_DSCH_OCT_Ad/2
  BMS_ALM_DSCH_OCT_Ad/1 -> BMS_ALM_DSCH_OCT_sat/1
  BMS_ALM_DSCH_OCT_sat/1 -> BMS_ALM_DSCH_OCT_Out/1
  Demux/4 -> BMS_ALM_DSCH_OCT_Sub/1(In1), BMS_ALM_DSCH_OCS_Sub/1(In1), BMS_ALM_CHRG_OCT_Sub/1(In1), BMS_ALM_BSU_OFFLINE_Sub/1(In1)
  BMS_ALM_DSCH_OCT_Sub/1(Out1) -> BMS_ALM_DSCH_OCT_Convert/1
  BMS_ALM_DSCH_OCT_Convert/1 -> BMS_ALM_DSCH_OCT_L/1
  BMS_ALM_DSCH_OCT_L/1 -> BMS_ALM_DSCH_OCT_S/1
  BMS_ALM_DSCH_OCT_S/1 -> BMS_ALM_DSCH_OCTcv/1
  BMS_ALM_DSCH_OCTcv/1 -> BMS_ALM_DSCH_OCT_F/1
  BMS_ALM_DSCH_OCS_F/1 -> BMS_ALM_DSCH_OCS_Ad/1
  BMS_ALM_DSCH_OCS_O/1 -> BMS_ALM_DSCH_OCS_Ad/2
  BMS_ALM_DSCH_OCS_Ad/1 -> BMS_ALM_DSCH_OCS_sat/1
  BMS_ALM_DSCH_OCS_sat/1 -> BMS_ALM_DSCH_OCS_Out/1
  BMS_ALM_DSCH_OCS_Sub/1(Out1) -> BMS_ALM_DSCH_OCS_Convert/1
  BMS_ALM_DSCH_OCS_Convert/1 -> BMS_ALM_DSCH_OCS_L/1
  BMS_ALM_DSCH_OCS_L/1 -> BMS_ALM_DSCH_OCS_S/1
  BMS_ALM_DSCH_OCS_S/1 -> BMS_ALM_DSCH_OCScv/1
  BMS_ALM_DSCH_OCScv/1 -> BMS_ALM_DSCH_OCS_F/1
  BMS_ALM_CHRG_OCT_F/1 -> BMS_ALM_CHRG_OCT_Ad/1
  BMS_ALM_CHRG_OCT_O/1 -> BMS_ALM_CHRG_OCT_Ad/2
  BMS_ALM_CHRG_OCT_Ad/1 -> BMS_ALM_CHRG_OCT_sat/1
  BMS_ALM_CHRG_OCT_sat/1 -> BMS_ALM_CHRG_OCT_Out/1
  BMS_ALM_CHRG_OCT_Sub/1(Out1) -> BMS_ALM_CHRG_OCT_Convert/1
  BMS_ALM_CHRG_OCT_Convert/1 -> BMS_ALM_CHRG_OCT_L/1
  BMS_ALM_CHRG_OCT_L/1 -> BMS_ALM_CHRG_OCT_S/1
  BMS_ALM_CHRG_OCT_S/1 -> BMS_ALM_CHRG_OCTcv/1
  BMS_ALM_CHRG_OCTcv/1 -> BMS_ALM_CHRG_OCT_F/1
  BMS_ALM_CHRG_OCS_F/1 -> BMS_ALM_CHRG_OCS_Ad/1
  BMS_ALM_CHRG_OCS_O/1 -> BMS_ALM_CHRG_OCS_Ad/2
  BMS_ALM_CHRG_OCS_Ad/1 -> BMS_ALM_CHRG_OCS_sat/1
  BMS_ALM_CHRG_OCS_sat/1 -> BMS_ALM_CHRG_OCS_Out/1
  Demux/3 -> BMS_ALM_BATT_UC_Sub/1(In1), BMS_ALM_BATT_OC_Sub/1(In1), BMS_ALM_BATT_UV_Sub/1(In1), BMS_ALM_CHRG_OCS_Sub/1(In1)
  BMS_ALM_CHRG_OCS_Sub/1(Out1) -> BMS_ALM_CHRG_OCS_Convert/1
  BMS_ALM_CHRG_OCS_Convert/1 -> BMS_ALM_CHRG_OCS_L/1
  BMS_ALM_CHRG_OCS_L/1 -> BMS_ALM_CHRG_OCS_S/1
  BMS_ALM_CHRG_OCS_S/1 -> BMS_ALM_CHRG_OCScv/1
  BMS_ALM_CHRG_OCScv/1 -> BMS_ALM_CHRG_OCS_F/1
  BMS_ALM_CELL_UV_F/1 -> BMS_ALM_CELL_UV_Ad/1
  BMS_ALM_CELL_UV_O/1 -> BMS_ALM_CELL_UV_Ad/2
  BMS_ALM_CELL_UV_Ad/1 -> BMS_ALM_CELL_UV_sat/1
  BMS_ALM_CELL_UV_sat/1 -> BMS_ALM_CELL_UV_Out/1
  Demux/1 -> BMS_ALM_CELL_OV_Sub/1(In1), BMS_ALM_CELL_OT_Sub/1(In1), BMS_ALM_CELL_UT_Sub/1(In1), BMS_ALM_CELL_UV_Sub/1(In1)
  BMS_ALM_CELL_UV_Sub/1(Out1) -> BMS_ALM_CELL_UV_Convert/1
  BMS_ALM_CELL_UV_Convert/1 -> BMS_ALM_CELL_UV_L/1
  BMS_ALM_CELL_UV_L/1 -> BMS_ALM_CELL_UV_S/1
  BMS_ALM_CELL_UV_S/1 -> BMS_ALM_CELL_UVcv/1
  BMS_ALM_CELL_UVcv/1 -> BMS_ALM_CELL_UV_F/1
  BMS_ALM_CELL_UT_F/1 -> BMS_ALM_CELL_UT_Ad/1
  BMS_ALM_CELL_UT_O/1 -> BMS_ALM_CELL_UT_Ad/2
  BMS_ALM_CELL_UT_Ad/1 -> BMS_ALM_CELL_UT_sat/1
  BMS_ALM_CELL_UT_sat/1 -> BMS_ALM_CELL_UT_Out/1
  BMS_ALM_CELL_UT_Sub/1(Out1) -> BMS_ALM_CELL_UT_Convert/1
  BMS_ALM_CELL_UT_Convert/1 -> BMS_ALM_CELL_UT_L/1
  BMS_ALM_CELL_UT_L/1 -> BMS_ALM_CELL_UT_S/1
  BMS_ALM_CELL_UT_S/1 -> BMS_ALM_CELL_UTcv/1
  BMS_ALM_CELL_UTcv/1 -> BMS_ALM_CELL_UT_F/1
  BMS_ALM_CELL_TBK_F/1 -> BMS_ALM_CELL_TBK_Ad/1
  BMS_ALM_CELL_TBK_O/1 -> BMS_ALM_CELL_TBK_Ad/2
  BMS_ALM_CELL_TBK_Ad/1 -> BMS_ALM_CELL_TBK_sat/1
  BMS_ALM_CELL_TBK_sat/1 -> BMS_ALM_CELL_TBK_Out/1
  Demux/2 -> BMS_ALM_CELL_DT_Sub/1(In1), BMS_ALM_BATT_OV_Sub/1(In1), BMS_ALM_CELL_DV_Sub/1(In1), BMS_ALM_CELL_LBK_Sub/1(In1), BMS_ALM_CELL_TBK_Sub/1(In1)
  BMS_ALM_CELL_TBK_Sub/1(Out1) -> BMS_ALM_CELL_TBK_Convert/1
  BMS_ALM_CELL_TBK_Convert/1 -> BMS_ALM_CELL_TBK_L/1
  BMS_ALM_CELL_TBK_L/1 -> BMS_ALM_CELL_TBK_S/1
  BMS_ALM_CELL_TBK_S/1 -> BMS_ALM_CELL_TBKcv/1
  BMS_ALM_CELL_TBKcv/1 -> BMS_ALM_CELL_TBK_F/1
  BMS_ALM_CELL_OV_F/1 -> BMS_ALM_CELL_OV_Ad/1
  BMS_ALM_CELL_OV_O/1 -> BMS_ALM_CELL_OV_Ad/2
  BMS_ALM_CELL_OV_Ad/1 -> BMS_ALM_CELL_OV_sat/1
  BMS_ALM_CELL_OV_sat/1 -> BMS_ALM_CELL_OV_Out/1
  BMS_ALM_CELL_OV_Sub/1(Out1) -> BMS_ALM_CELL_OV_Convert/1
  BMS_ALM_CELL_OV_Convert/1 -> BMS_ALM_CELL_OV_L/1
  BMS_ALM_CELL_OV_L/1 -> BMS_ALM_CELL_OV_S/1
  BMS_ALM_CELL_OV_S/1 -> BMS_ALM_CELL_OVcv/1
  BMS_ALM_CELL_OVcv/1 -> BMS_ALM_CELL_OV_F/1
  BMS_ALM_CELL_OT_F/1 -> BMS_ALM_CELL_OT_Ad/1
  BMS_ALM_CELL_OT_O/1 -> BMS_ALM_CELL_OT_Ad/2
  BMS_ALM_CELL_OT_Ad/1 -> BMS_ALM_CELL_OT_sat/1
  BMS_ALM_CELL_OT_sat/1 -> BMS_ALM_CELL_OT_Out/1
  BMS_ALM_CELL_OT_Sub/1(Out1) -> BMS_ALM_CELL_OT_Convert/1
  BMS_ALM_CELL_OT_Convert/1 -> BMS_ALM_CELL_OT_L/1
  BMS_ALM_CELL_OT_L/1 -> BMS_ALM_CELL_OT_S/1
  BMS_ALM_CELL_OT_S/1 -> BMS_ALM_CELL_OTcv/1
  BMS_ALM_CELL_OTcv/1 -> BMS_ALM_CELL_OT_F/1
  BMS_ALM_CELL_LBK_F/1 -> BMS_ALM_CELL_LBK_Ad/1
  BMS_ALM_CELL_LBK_O/1 -> BMS_ALM_CELL_LBK_Ad/2
  BMS_ALM_CELL_LBK_Ad/1 -> BMS_ALM_CELL_LBK_sat/1
  BMS_ALM_CELL_LBK_sat/1 -> BMS_ALM_CELL_LBK_Out/1
  BMS_ALM_CELL_LBK_Sub/1(Out1) -> BMS_ALM_CELL_LBK_Convert/1
  BMS_ALM_CELL_LBK_Convert/1 -> BMS_ALM_CELL_LBK_L/1
  BMS_ALM_CELL_LBK_L/1 -> BMS_ALM_CELL_LBK_S/1
  BMS_ALM_CELL_LBK_S/1 -> BMS_ALM_CELL_LBKcv/1
  BMS_ALM_CELL_LBKcv/1 -> BMS_ALM_CELL_LBK_F/1
  BMS_ALM_CELL_DV_F/1 -> BMS_ALM_CELL_DV_Ad/1
  BMS_ALM_CELL_DV_O/1 -> BMS_ALM_CELL_DV_Ad/2
  BMS_ALM_CELL_DV_Ad/1 -> BMS_ALM_CELL_DV_sat/1
  BMS_ALM_CELL_DV_sat/1 -> BMS_ALM_CELL_DV_Out/1
  BMS_ALM_CELL_DV_Sub/1(Out1) -> BMS_ALM_CELL_DV_Convert/1
  BMS_ALM_CELL_DV_Convert/1 -> BMS_ALM_CELL_DV_L/1
  BMS_ALM_CELL_DV_L/1 -> BMS_ALM_CELL_DV_S/1
  BMS_ALM_CELL_DV_S/1 -> BMS_ALM_CELL_DVcv/1
  BMS_ALM_CELL_DVcv/1 -> BMS_ALM_CELL_DV_F/1
  BMS_ALM_CELL_DT_F/1 -> BMS_ALM_CELL_DT_Ad/1
  BMS_ALM_CELL_DT_O/1 -> BMS_ALM_CELL_DT_Ad/2
  BMS_ALM_CELL_DT_Ad/1 -> BMS_ALM_CELL_DT_sat/1
  BMS_ALM_CELL_DT_sat/1 -> BMS_ALM_CELL_DT_Out/1
  BMS_ALM_CELL_DT_Sub/1(Out1) -> BMS_ALM_CELL_DT_Convert/1
  BMS_ALM_CELL_DT_Convert/1 -> BMS_ALM_CELL_DT_L/1
  BMS_ALM_CELL_DT_L/1 -> BMS_ALM_CELL_DT_S/1
  BMS_ALM_CELL_DT_S/1 -> BMS_ALM_CELL_DTcv/1
  BMS_ALM_CELL_DTcv/1 -> BMS_ALM_CELL_DT_F/1
  BMS_ALM_BSU_OFFLINE_F/1 -> BMS_ALM_BSU_OFFLINE_Ad/1
  BMS_ALM_BSU_OFFLINE_O/1 -> BMS_ALM_BSU_OFFLINE_Ad/2
  BMS_ALM_BSU_OFFLINE_Ad/1 -> BMS_ALM_BSU_OFFLINE_sat/1
  BMS_ALM_BSU_OFFLINE_sat/1 -> BMS_ALM_BSU_OFFLINE_Out/1
  BMS_ALM_BSU_OFFLINE_Sub/1(Out1) -> BMS_ALM_BSU_OFFLINE_Convert/1
  BMS_ALM_BSU_OFFLINE_Convert/1 -> BMS_ALM_BSU_OFFLINE_L/1
  BMS_ALM_BSU_OFFLINE_L/1 -> BMS_ALM_BSU_OFFLINE_S/1
  BMS_ALM_BSU_OFFLINE_S/1 -> BMS_ALM_BSU_OFFLINEcv/1
  BMS_ALM_BSU_OFFLINEcv/1 -> BMS_ALM_BSU_OFFLINE_F/1
  BMS_ALM_BSU_FAULT_F/1 -> BMS_ALM_BSU_FAULT_Ad/1
  BMS_ALM_BSU_FAULT_O/1 -> BMS_ALM_BSU_FAULT_Ad/2
  BMS_ALM_BSU_FAULT_Ad/1 -> BMS_ALM_BSU_FAULT_sat/1
  BMS_ALM_BSU_FAULT_sat/1 -> BMS_ALM_BSU_FAULT_Out/1
  BMS_ALM_BSU_FAULT_Sub/1(Out1) -> BMS_ALM_BSU_FAULT_Convert/1
  BMS_ALM_BSU_FAULT_Convert/1 -> BMS_ALM_BSU_FAULT_L/1
  BMS_ALM_BSU_FAULT_L/1 -> BMS_ALM_BSU_FAULT_S/1
  BMS_ALM_BSU_FAULT_S/1 -> BMS_ALM_BSU_FAULTcv/1
  BMS_ALM_BSU_FAULTcv/1 -> BMS_ALM_BSU_FAULT_F/1
  BMS_ALM_BMU_FAIL_F/1 -> BMS_ALM_BMU_FAIL_Ad/1
  BMS_ALM_BMU_FAIL_O/1 -> BMS_ALM_BMU_FAIL_Ad/2
  BMS_ALM_BMU_FAIL_Ad/1 -> BMS_ALM_BMU_FAIL_sat/1
  BMS_ALM_BMU_FAIL_sat/1 -> BMS_ALM_BMU_FAIL_Out/1
  BMS_ALM_BMU_FAIL_Sub/1(Out1) -> BMS_ALM_BMU_FAIL_Convert/1
  BMS_ALM_BMU_FAIL_Convert/1 -> BMS_ALM_BMU_FAIL_L/1
  BMS_ALM_BMU_FAIL_L/1 -> BMS_ALM_BMU_FAIL_S/1
  BMS_ALM_BMU_FAIL_S/1 -> BMS_ALM_BMU_FAILcv/1
  BMS_ALM_BMU_FAILcv/1 -> BMS_ALM_BMU_FAIL_F/1
  BMS_ALM_BATT_UV_F/1 -> BMS_ALM_BATT_UV_Ad/1
  BMS_ALM_BATT_UV_O/1 -> BMS_ALM_BATT_UV_Ad/2
  BMS_ALM_BATT_UV_Ad/1 -> BMS_ALM_BATT_UV_sat/1
  BMS_ALM_BATT_UV_sat/1 -> BMS_ALM_BATT_UV_Out/1
  BMS_ALM_BATT_UV_Sub/1(Out1) -> BMS_ALM_BATT_UV_Convert/1
  BMS_ALM_BATT_UV_Convert/1 -> BMS_ALM_BATT_UV_L/1
  BMS_ALM_BATT_UV_L/1 -> BMS_ALM_BATT_UV_S/1
  BMS_ALM_BATT_UV_S/1 -> BMS_ALM_BATT_UVcv/1
  BMS_ALM_BATT_UVcv/1 -> BMS_ALM_BATT_UV_F/1
  BMS_ALM_BATT_UC_F/1 -> BMS_ALM_BATT_UC_Ad/1
  BMS_ALM_BATT_UC_O/1 -> BMS_ALM_BATT_UC_Ad/2
  BMS_ALM_BATT_UC_Ad/1 -> BMS_ALM_BATT_UC_sat/1
  BMS_ALM_BATT_UC_sat/1 -> BMS_ALM_BATT_UC_Out/1
  BMS_ALM_BATT_UC_Sub/1(Out1) -> BMS_ALM_BATT_UC_Convert/1
  BMS_ALM_BATT_UC_Convert/1 -> BMS_ALM_BATT_UC_L/1
  BMS_ALM_BATT_UC_L/1 -> BMS_ALM_BATT_UC_S/1
  BMS_ALM_BATT_UC_S/1 -> BMS_ALM_BATT_UCcv/1
  BMS_ALM_BATT_UCcv/1 -> BMS_ALM_BATT_UC_F/1
  BMS_ALM_BATT_OV_F/1 -> BMS_ALM_BATT_OV_Ad/1
  BMS_ALM_BATT_OV_O/1 -> BMS_ALM_BATT_OV_Ad/2
  BMS_ALM_BATT_OV_Ad/1 -> BMS_ALM_BATT_OV_sat/1
  BMS_ALM_BATT_OV_sat/1 -> BMS_ALM_BATT_OV_Out/1
  BMS_ALM_BATT_OV_Sub/1(Out1) -> BMS_ALM_BATT_OV_Convert/1
  BMS_ALM_BATT_OV_Convert/1 -> BMS_ALM_BATT_OV_L/1
  BMS_ALM_BATT_OV_L/1 -> BMS_ALM_BATT_OV_S/1
  BMS_ALM_BATT_OV_S/1 -> BMS_ALM_BATT_OVcv/1
  BMS_ALM_BATT_OVcv/1 -> BMS_ALM_BATT_OV_F/1
  BMS_ALM_BATT_OC_F/1 -> BMS_ALM_BATT_OC_Ad/1
  BMS_ALM_BATT_OC_O/1 -> BMS_ALM_BATT_OC_Ad/2
  BMS_ALM_BATT_OC_Ad/1 -> BMS_ALM_BATT_OC_sat/1
  BMS_ALM_BATT_OC_sat/1 -> BMS_ALM_BATT_OC_Out/1
  BMS_ALM_BATT_OC_Sub/1(Out1) -> BMS_ALM_BATT_OC_Convert/1
  BMS_ALM_BATT_OC_Convert/1 -> BMS_ALM_BATT_OC_L/1
  BMS_ALM_BATT_OC_L/1 -> BMS_ALM_BATT_OC_S/1
  BMS_ALM_BATT_OC_S/1 -> BMS_ALM_BATT_OCcv/1
  BMS_ALM_BATT_OCcv/1 -> BMS_ALM_BATT_OC_F/1
  BMS_ALM_AUX_FAIL_F/1 -> BMS_ALM_AUX_FAIL_Ad/1
  BMS_ALM_AUX_FAIL_O/1 -> BMS_ALM_AUX_FAIL_Ad/2
  BMS_ALM_AUX_FAIL_Ad/1 -> BMS_ALM_AUX_FAIL_sat/1
  BMS_ALM_AUX_FAIL_sat/1 -> BMS_ALM_AUX_FAIL_Out/1
  BMS_ALM_AUX_FAIL_Sub/1(Out1) -> BMS_ALM_AUX_FAIL_Convert/1
  BMS_ALM_AUX_FAIL_Convert/1 -> BMS_ALM_AUX_FAIL_L/1
  BMS_ALM_AUX_FAIL_L/1 -> BMS_ALM_AUX_FAIL_S/1
  BMS_ALM_AUX_FAIL_S/1 -> BMS_ALM_AUX_FAILcv/1
  BMS_ALM_AUX_FAILcv/1 -> BMS_ALM_AUX_FAIL_F/1
  input/1 -> Demux/1
  Demux/7 -> Terminator/1
  Demux/8 -> Terminator1/1

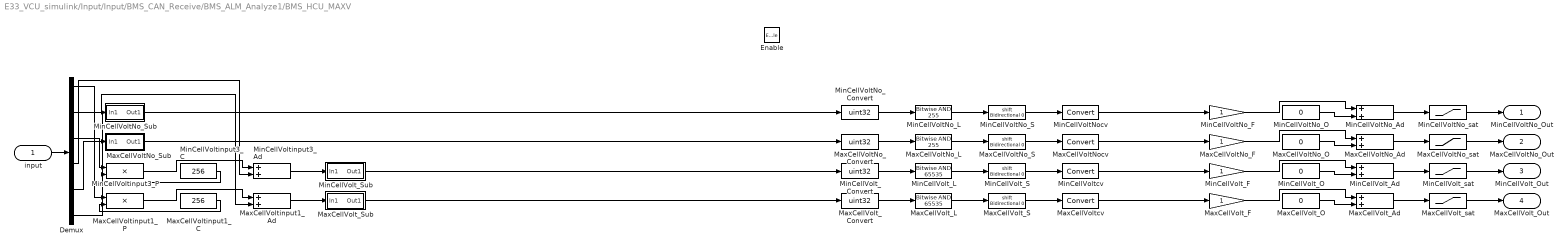
== system E33_VCU_simulink/Input/Input/BMS_CAN_Receive/BMS_ALM_Analyze1/BMS_HCU_MAXV ==
  input : Inport
  Enable : EnablePort
  Demux : Demux  Outputs=6
  MaxCellVoltNo_Ad : Sum
  MaxCellVoltNo_Convert : DataTypeConversion  OutDataTypeStr=uint32
  MaxCellVoltNo_F : Gain
  MaxCellVoltNo_L : simulink/Logic and Bit Operations/Bitwise Operator  logicop=AND  UseBitMask=on  BitMask=255  BitMaskRealWorld=Stored Integer
  MaxCellVoltNo_O : Constant  Value=0  OutDataTypeStr=single
  MaxCellVoltNo_S : ArithShift
  MaxCellVoltNo_Sub : Subsystem
  MaxCellVoltNo_sat : Saturate  UpperLimit=255  LowerLimit=0
  MaxCellVoltNocv : DataTypeConversion
  MaxCellVolt_Ad : Sum
  MaxCellVolt_Convert : DataTypeConversion  OutDataTypeStr=uint32
  MaxCellVolt_F : Gain
  MaxCellVolt_L : simulink/Logic and Bit Operations/Bitwise Operator  logicop=AND  UseBitMask=on  BitMask=65535  BitMaskRealWorld=Stored Integer
  MaxCellVolt_O : Constant  Value=0  OutDataTypeStr=single
  MaxCellVolt_S : ArithShift
  MaxCellVolt_Sub : Subsystem
  MaxCellVolt_sat : Saturate  UpperLimit=5000  LowerLimit=0
  MaxCellVoltcv : DataTypeConversion
  MaxCellVoltinput1_Ad : Sum
  MaxCellVoltinput1_C : Constant  Value=256
  MaxCellVoltinput1_P : Product
  MinCellVoltNo_Ad : Sum
  MinCellVoltNo_Convert : DataTypeConversion  OutDataTypeStr=uint32
  MinCellVoltNo_F : Gain
  MinCellVoltNo_L : simulink/Logic and Bit Operations/Bitwise Operator  logicop=AND  UseBitMask=on  BitMask=255  BitMaskRealWorld=Stored Integer
  MinCellVoltNo_O : Constant  Value=0  OutDataTypeStr=single
  MinCellVoltNo_S : ArithShift
  MinCellVoltNo_Sub : Subsystem
  MinCellVoltNo_sat : Saturate  UpperLimit=255  LowerLimit=0
  MinCellVoltNocv : DataTypeConversion
  MinCellVolt_Ad : Sum
  MinCellVolt_Convert : DataTypeConversion  OutDataTypeStr=uint32
  MinCellVolt_F : Gain
  MinCellVolt_L : simulink/Logic and Bit Operations/Bitwise Operator  logicop=AND  UseBitMask=on  BitMask=65535  BitMaskRealWorld=Stored Integer
  MinCellVolt_O : Constant  Value=0  OutDataTypeStr=single
  MinCellVolt_S : ArithShift
  MinCellVolt_Sub : Subsystem
  MinCellVolt_sat : Saturate  UpperLimit=5000  LowerLimit=0
  MinCellVoltcv : DataTypeConversion
  MinCellVoltinput3_Ad : Sum
  MinCellVoltinput3_C : Constant  Value=256
  MinCellVoltinput3_P : Product
  MinCellVoltNo_Out : Outport
  MaxCellVoltNo_Out : Outport  Port=2
  MinCellVolt_Out : Outport  Port=3
  MaxCellVolt_Out : Outport  Port=4
  wires:
  MinCellVoltNo_F/1 -> MinCellVoltNo_Ad/1
  MinCellVoltNo_O/1 -> MinCellVoltNo_Ad/2
  MinCellVoltNo_Ad/1 -> MinCellVoltNo_sat/1
  MinCellVoltNo_sat/1 -> MinCellVoltNo_Out/1
  Demux/6 -> MinCellVoltNo_Sub/1(In1)
  MinCellVoltNo_Sub/1(Out1) -> MinCellVoltNo_Convert/1
  MinCellVoltNo_Convert/1 -> MinCellVoltNo_L/1
  MinCellVoltNo_L/1 -> MinCellVoltNo_S/1
  MinCellVoltNo_S/1 -> MinCellVoltNocv/1
  MinCellVoltNocv/1 -> MinCellVoltNo_F/1
  MaxCellVoltNo_F/1 -> MaxCellVoltNo_Ad/1
  MaxCellVoltNo_O/1 -> MaxCellVoltNo_Ad/2
  MaxCellVoltNo_Ad/1 -> MaxCellVoltNo_sat/1
  MaxCellVoltNo_sat/1 -> MaxCellVoltNo_Out/1
  Demux/5 -> MaxCellVoltNo_Sub/1(In1)
  MaxCellVoltNo_Sub/1(Out1) -> MaxCellVoltNo_Convert/1
  MaxCellVoltNo_Convert/1 -> MaxCellVoltNo_L/1
  MaxCellVoltNo_L/1 -> MaxCellVoltNo_S/1
  MaxCellVoltNo_S/1 -> MaxCellVoltNocv/1
  MaxCellVoltNocv/1 -> MaxCellVoltNo_F/1
  MinCellVolt_F/1 -> MinCellVolt_Ad/1
  MinCellVolt_O/1 -> MinCellVolt_Ad/2
  MinCellVolt_Ad/1 -> MinCellVolt_sat/1
  MinCellVolt_sat/1 -> MinCellVolt_Out/1
  Demux/3 -> MinCellVoltinput3_P/1
  MinCellVoltinput3_C/1 -> MinCellVoltinput3_P/2
  MinCellVoltinput3_P/1 -> MinCellVoltinput3_Ad/1
  Demux/4 -> MinCellVoltinput3_Ad/2
  MinCellVoltinput3_Ad/1 -> MinCellVolt_Sub/1(In1)
  MinCellVolt_Sub/1(Out1) -> MinCellVolt_Convert/1
  MinCellVolt_Convert/1 -> MinCellVolt_L/1
  MinCellVolt_L/1 -> MinCellVolt_S/1
  MinCellVolt_S/1 -> MinCellVoltcv/1
  MinCellVoltcv/1 -> MinCellVolt_F/1
  MaxCellVolt_F/1 -> MaxCellVolt_Ad/1
  MaxCellVolt_O/1 -> MaxCellVolt_Ad/2
  MaxCellVolt_Ad/1 -> MaxCellVolt_sat/1
  MaxCellVolt_sat/1 -> MaxCellVolt_Out/1
  Demux/1 -> MaxCellVoltinput1_P/1
  MaxCellVoltinput1_C/1 -> MaxCellVoltinput1_P/2
  MaxCellVoltinput1_P/1 -> MaxCellVoltinput1_Ad/1
  Demux/2 -> MaxCellVoltinput1_Ad/2
  MaxCellVoltinput1_Ad/1 -> MaxCellVolt_Sub/1(In1)
  MaxCellVolt_Sub/1(Out1) -> MaxCellVolt_Convert/1
  MaxCellVolt_Convert/1 -> MaxCellVolt_L/1
  MaxCellVolt_L/1 -> MaxCellVolt_S/1
  MaxCellVolt_S/1 -> MaxCellVoltcv/1
  MaxCellVoltcv/1 -> MaxCellVolt_F/1
  input/1 -> Demux/1
